simulink model "project_2"  (R2020b)
settings: Solver=VariableStepAuto  StartTime=0.0  StopTime=10.0  RelTol=1e-3
settings Model: Creator=shrin  LastModifiedBy=shrin

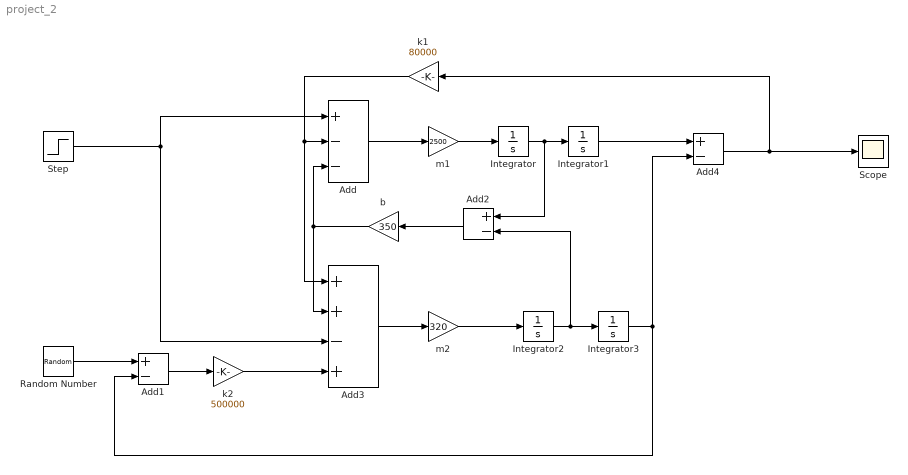
== system project_2 ==
  Add : Sum  Inputs=+--
  Add1 : Sum  Inputs=+-
  Add2 : Sum  Inputs=+-
  Add3 : Sum  Inputs=++-+
  Add4 : Sum  Inputs=+-
  Integrator{,1..3} (4 alike) : Integrator
  Random Number : RandomNumber  SampleTime=0.1
  Scope : Scope
  Step : Step  SampleTime=0
  b : Gain  Gain=350
  k1 : Gain  Gain=80000
  k2 : Gain  Gain=500000
  m1 : Gain  Gain=2500
  m2 : Gain  Gain=320
  wires:
  Random Number/1 -> Add1/1
  Add1/1 -> k2/1
  Step/1 -> Add3/3, Add/1
  k2/1 -> Add3/4
  Add/1 -> m1/1
  m1/1 -> Integrator/1
  Integrator/1 -> Add2/1, Integrator1/1
  Integrator1/1 -> Add4/1
  Add4/1 -> k1/1, Scope/1
  m2/1 -> Integrator2/1
  Integrator2/1 -> Add2/2, Integrator3/1
  Integrator3/1 -> Add4/2, Add1/2
  Add2/1 -> b/1
  b/1 -> Add3/2, Add/3
  k1/1 -> Add3/1, Add/2
  Add3/1 -> m2/1
